simulink model "PhysicsBased_Tutorials"  (R2021a)
settings: Solver=FixedStepAuto  StartTime=0.0  StopTime=50  FixedStep=.0015  RelTol=1e-3
undefined symbols (not defined in the file): Ion, Li
libraries: PB_Library_Master x57, Lib_Solve_SSNRSolverJC_EMTAT x6, Lib_Solve_SSNRSolverJC_TMATS x1, TemperatureBlock x1
(part 1 of 2)
settings Model: Creator=nbutler2  LastModifiedBy=sfaulk
settings SolverCC: AlgebraicLoopSolver=TrustRegion
settings DebuggingCC: SFMachineParentedDataDiag=warning

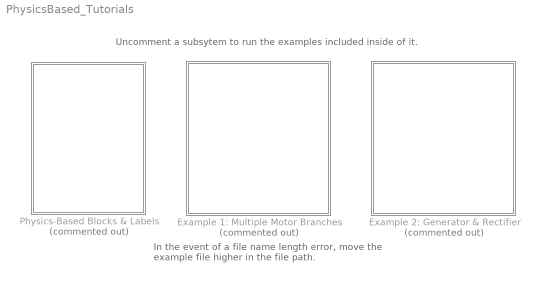
== system PhysicsBased_Tutorials ==
  note: Uncomment a subsytem to run the examples included inside of it.
  note: In the event of a file name length error, move the example file higher in the file path.
  Example 1: Multiple Motor Branches : Subsystem  Commented=on
  Example 2: Generator & Rectifier : Subsystem  Commented=on
  Physics-Based Blocks & Labels : Subsystem  Commented=on

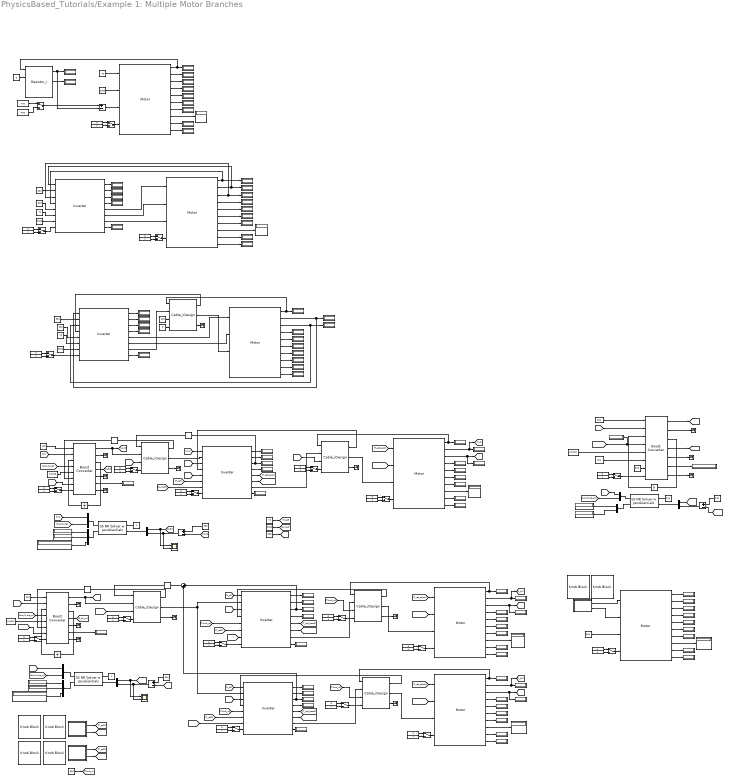
== system PhysicsBased_Tutorials/Example 1: Multiple Motor Branches ==
  note: ------------------------------------------------
      | Created by Nathan Butler
      | NASA Glenn Research Center
      | MATLAB R2020b
      | Spring 2021
      | ------------------------------------------------
  note: Current Error
  note: Solver finds solution for current input and duty cycle by driving power error (P_Err) to 0 and Vout to desired output voltage (Vdesired-Vout = 0).
  note: Model 4A: Boost Converter Example
  note: For a more detailed example, see:
      | EMTAT->Examples->Physics Based->BoostConverter_Example.m
  note: Model Inputs
  note: V_s & PF sent to inverter
  note: Some general inputs
  note: This example adds the boost converter component to the above model. A solver is used to solve for the input current and duty cycle for the boost converter. Notice that current demand is still sent backwards throughout the circuit and voltage is sent forwards.
  note: Similar to example above, but now includes cable with some small voltage loss. This example shows how the cable component can be incorporated into systems.
  note: Motor 3: Inverter-Cable-Motor Example
  note: Model 1: Current-Based Resistor-Motor Example
  note: Solves for Boost Converter input current (Iin) and duty cycle by driving P_err to zero and Vout to desired output voltage of 550V.
  note: Model includes Inverter and AC Motor. Inverter takes DC voltage input (V_batt) along with required inputs (V_s, PF, I_RMS) from motor and outputs power and current requirements (P_in_inv, I_In_inv). Mechanical properties and V_batt are passed through inverter to motor.
  note: Multi-Branch Motor Example
  note: Model 5A: Motor with Control Knobs
  note: <--- Current demanded sent backwards along top of model <---
  note: Model 4B: BoostConv-Inverter-Motor-withCables Branch
  note: Model 2: Inverter-Motor Example
  note: DC to AC
  note: DC to AC
  note: Set to desired output voltage (set point)
      | From iDesign mask window
  note: ---> Voltage sent forwards through model --->
  note: ---> Voltage sent forwards through model --->
  note: DC to AC
  note: <--- Current demanded sent backwards along top of model <---
  note: V_s & PF sent to inverter
  note: Solves for Boost Converter input current (Iin) and duty cycle by driving P_err to zero and Vout to desired output voltage of 550V.
  note: Set to desired output voltage (set point)
      | From iDesign mask window
  note: Model 5B: Multiple Motor Branch Example
  note: DC to AC
  note: DC to AC
  note: V_s & PF sent to inverter
  note: Set to:
      | (load power)/(voltage output)
      | From iDesign mask window
  note: Set to:
      | (min Vin + max Vin)/2
      | From iDesign mask window
  note: WORKS BEST WITH FIXED
      | STEP SIZE SOLVER. ENSURE
      | STEP SIZE AGREES WITH INPUT
      | TO dt ON BOOST CONVERTER
  note: Set to desired output voltage (set point)
      | From iDesign mask window
  note: Voltage Error
  note: Power Error
  note: Voltage Error
  note: Power Error
  note: Current Error
  note: Voltage Error
  note: Power Error
  note: Current Error
  note: Voltage Error
  note: Power Error
  note: Current Error
  note: Voltage Error
  note: Power Error
  note: Current Error
  note: Fault Toggle:
      | 0 is unfaulted
      | 1 is fault
  note: Fault Toggle:
      | 0 is unfaulted
      | 1 is fault
  note: Fault Toggle:
      | 0 is unfaulted
      | 1 is fault
  note: Fault Toggle:
      | 0 is unfaulted
      | 1 is fault
  note: Fault Toggle:
      | 0 is unfaulted
      | 1 is fault
  note: Fault Toggle:
      | 0 is unfaulted
      | 1 is fault
  note: Fault Toggle:
      | 0 is unfaulted
      | 1 is fault
  note: Fault Toggle:
      | 0 is unfaulted
      | 1 is fault
  note: Fault Toggle:
      | 0 is unfaulted
      | 1 is fault
  Add1 : Sum  Inputs=+-
  Add2 : Sum  Inputs=+-
  Add3 : Sum  Inputs=+-
  Boost Converter : PB_Library_Master/Boost Converter  Pdis_M=1  C_M=1.65e-07  L_M=1.7399e-05  Ron_M=0.0012  RC_M=0.037475  RL_M=0.0057739  QgTotal_M=8.6e-07  Vdiode_M=1.4  TRise_M=2.2e-08  TFall_M=8e-09  Fsw_M=250000  Vgate_M=3.5  n_MOSFET=2  MassEst_M=82.533  TempIn=Celsius  vOut=550  pow=22000  minV=110  maxV=130  rippleMode=Use defaults (5% of voltage output and 10% of inductor current)  vRip=.05  iRip=.1  freqMode=Use default frequency (250 kHz)  freq=250e3
  Boost Converter1 : PB_Library_Master/Boost Converter  Pdis_M=1  C_M=1.65e-07  L_M=1.7804e-05  Ron_M=0.0012  RC_M=0.037475  RL_M=0.0057739  QgTotal_M=8.6e-07  Vdiode_M=1.4  TRise_M=2.2e-08  TFall_M=8e-09  Fsw_M=250000  Vgate_M=3.5  n_MOSFET=2  MassEst_M=82.533  TempIn=Celsius  vOut=600  pow=22000  minV=110  maxV=130  rippleMode=Use defaults (5% of voltage output and 10% of inductor current)  vRip=.05  iRip=.1  freqMode=Use default frequency (250 kHz)  freq=250e3
  Boost Converter2 : PB_Library_Master/Boost Converter  Pdis_M=1  C_M=1.65e-07  L_M=0.00011412  Ron_M=0.0092  RC_M=0.037475  RL_M=0.03635  QgTotal_M=7.4e-08  Vdiode_M=1.4  TRise_M=7e-09  TFall_M=1e-08  Fsw_M=250000  Vgate_M=3.5  n_MOSFET=1  MassEst_M=37.515  TempIn=Celsius  vOut=540  pow=10000  minV=240  maxV=260  rippleMode=Use defaults (5% of voltage output and 10% of inductor current)  vRip=.05  iRip=.1  freqMode=Use default frequency (250 kHz)  freq=250e3
  Bus Selector1 : BusSelector  OutputSignals=Converged,JacFailed,J
  Bus Selector2 : BusSelector  OutputSignals=Converged,JacFailed,J
  Bus Selector3 : BusSelector  OutputSignals=Converged,JacFailed
  Cable_iDesign{,1..5} (6 alike) : PB_Library_Master/Cable_iDesign  rad_c_M=0.94407  t_i_M=1.0013  Mass_M=159.0996  R_init=0.006  alpha=0.00393  V_in=120  V_drop=.3  I_out=40  Len=100  FS=1.5  Mat_c=Copper  UResis=0  UDens_C=0  UAlpha=0  Mat_i=PVC  UDens_I=0  UEpsilon=0
  Constant{,5,9,14,25,42} (6 alike) : Constant  Value=528
  Constant{1,7,20,26} (4 alike) : Constant  Value=70
  Constant10 : Constant  Value=true
  Constant11 : Constant  Value=250  VectorParams1D=off  SampleTime=-1
  Constant12 : Constant  Value=120
  Constant{13,15,17,19,27,29,31,33,35,37,41,45,47,50,52,54,57,60,62,65,67} (21 alike) : Constant
  Constant16 : Constant  Value=0.0015  VectorParams1D=off
  Constant18 : Constant  Value=600
  Constant{2,8,21,39} (4 alike) : Constant  Value=3000
  Constant22 : Constant  Value=150
  Constant23 : Constant  Value=0.0015  VectorParams1D=off
  Constant{4,24,38,46} (4 alike) : Constant  Value=550
  Constant{6,28,30,32,34,36,43,48..49,51,53,55..56,58..59,61,63..64,66,68} (20 alike) : Constant  Value=0
  Constant3 : Constant  Value=5
  Constant40 : Constant  Value=120
  Constant44 : Constant  Value=0.0015  VectorParams1D=off
  Current_Final : Display
  Current_Final1 : Display
  Demux : Demux  Outputs=2
  Demux1 : Demux  Outputs=2
  Demux2 : Demux  Outputs=2
  Desired Vout : Constant  Value=540
  Display{,1..19,22..43,53..60,63..82,85..110,113..117,128..133} (107 alike) : Display
  Integrator1 : Integrator
  Integrator2 : Integrator
  Integrator3 : Integrator  InitialCondition=[0;0]
  Inverter{,1..4} (5 alike) : PB_Library_Master/Inverter  T_M=[25 175]  u_D_M=[1.16666666666667 0.999999999999998]  u_ce0_M=[0.971428571428571 0.848275862068965]  R_c_M=[0.0285714285714286 0.0551724137931034]  R_D_M=[0.0238095238095238 0.0294117647058824]  E0_M=[6.00000000000002e-05 6.00000000000002e-05]  E1_M=[5.6e-05 5.6e-05]  f_sw_M=20000  L_s_M=0.1  P_max_I=22000  V_phase_I=600  f_sw_I=0  L_s_I=0.1
  Knob : KnobBlock  ScaleMax=80
  Knob1 : KnobBlock  ScaleMax=3000
  Knob2 : KnobBlock  ScaleMax=80
  Knob3 : KnobBlock  ScaleMax=3000
  Knob4 : KnobBlock  ScaleMax=80
  Knob5 : KnobBlock  ScaleMax=3000
  Manual Switch{,1..19} (20 alike) : ManualSwitch
  Memory{1..4} (4 alike) : Memory
  Motor{,1..6} (7 alike) : PB_Library_Master/Motor  pp=2.5  flux_m=0.46219  R_s=0.032  L_s=0.00115  P_Fe_Nom=904.3614  S_nom=3000  T_nom=70  P_out_max=22000  I_max=36.5  P_in_max=30000  T_max=80  MassEst_M=136.5892  Poles_i=5  R_s_i=.032  L_s_i=.00086+0.00029  S_nom_i=3000  T_nom_i=70  P_out_max_i=22000  I_max_i=36.5  P_in_max_i=30000  K_i=121  V_nom_i=368  T_max_i=80  CalculatePFe=Compute iron losses automatically  P_Fe_Nom_i=0  I_nom_i=36.5  PF_nom_i=0.99  P_Fe_Calc_Flag=1
  Motor 1 Control : Subsystem  mask{T_ref=71.10092157679236, S_mech=2953.766794958315}
      mask Display:
      | port_label('output', 1, 'T_ref');
      | port_label('output', 2, 'S_mech');
  Motor 2 Control : Subsystem  mask{T_ref=40.40733620046448, S_mech=2126.86052952404}
      mask Display:
      | port_label('output', 1, 'T_ref');
      | port_label('output', 2, 'S_mech');
  Mux : Mux  Inputs=2
  Mux1 : Mux  Inputs=2
  Mux2 : Mux  Inputs=2
  Resistor_I : PB_Library_Master/Resistor_I  TempIn=Celsius
  SS NR Solver w JacobianCalc : Lib_Solve_SSNRSolverJC_EMTAT/SS NR Solver w JacobianCalc  SJac_Per_M=.01 * [1 -1; 1 -1]  SNR_IC_M=[1;.5]  SNR_DX_M=10  SNR_Mx_M=[100000;.99999]  SNR_Mn_M=[0.00001;.0001]  SJacobianAttempts_M=200  Cond_Limits_M=0.0001
  SS NR Solver w JacobianCalc1 : Lib_Solve_SSNRSolverJC_EMTAT/SS NR Solver w JacobianCalc  SJac_Per_M=.01 * [1 -1; 1 -1]  SNR_IC_M=[1;.5]  SNR_DX_M=10  SNR_Mx_M=[100000;.99999]  SNR_Mn_M=[0.00001;.0001]  SJacobianAttempts_M=200  Cond_Limits_M=0.0001
  SS NR Solver w JacobianCalc3 : Lib_Solve_SSNRSolverJC_EMTAT/SS NR Solver w JacobianCalc  SJac_Per_M=.01 * [1 -1; 1 -1]  SNR_IC_M=[1;.5]  SNR_DX_M=10  SNR_Mx_M=[100000;.99999]  SNR_Mn_M=[0.00001;.0001]  SJacobianAttempts_M=200  Cond_Limits_M=0.0001
  Scope1 : Scope  NumInputPorts=2
  Scope2 : Scope  NumInputPorts=2
  Subsystem5 : Subsystem  mask{T_ref=78.74341928710747, S_mech=2893.268008214925}
      mask Display:
      | port_label('output', 1, 'T_ref');
      | port_label('output', 2, 'S_mech');
  Subtract : Sum  Inputs=+-
  Sum1 : Sum  Inputs=|++
  Terminator{,1..14} (15 alike) : Terminator
  V From Source : Constant  Value=700
  V From Source1 : Constant  Value=400
  wires:
  Inverter/4 -> Display37/1
  Constant25/1 -> Inverter/5
  [S_mech] -> Inverter2/7
  Subsystem5/1(Out1) -> Motor6/1
  Inverter2/3 -> Memory1/1, Display80/1  "Current demanded by inverter is input to cable"
  Cable_iDesign3/1 -> Inverter2/4  "Current demanded by cable is input to inverter"
  Constant24/1 -> Inverter/2
  Inverter/5 -> Motor1/1  "Torque passed through inverter to motor"
  Inverter/2 -> Display39/1
  Boost Converter/1 -> Cable_iDesign2/2, [Vout]  "V from Boost Converter"
  Bus Selector1/3 -> Display98/1  "<J>"
  Inverter2/4 -> Display79/1
  [S_mech_pass] -> Motor3/2
  Motor1/1 -> Inverter/4, Display77/1  "Current demanded by motor is input to previous block"
  Constant42/1 -> [TAmb]
  Constant38/1 -> Motor6/3
  [TAmb] -> Cable_iDesign3/3
  [dutyCycle] -> Boost Converter/4
  Inverter/1 -> Display40/1
  Constant20/1 -> Inverter/6
  Boost Converter/5 -> Terminator6/1
  Bus Selector1/2 -> Display97/1  "<JacFailed>"
  Memory2/1 -> Boost Converter/6  "Current demanded by cable is input into boost converter"
  Cable_iDesign2/3 -> Terminator3/1
  SS NR Solver w JacobianCalc1/1 -> Demux/1
  Inverter/8 -> Display36/1
  Motor3/2 -> [V_s], Display93/1
  Inverter/3 -> Display38/1
  Motor1/3 -> Inverter/3, Display75/1  "Power Factor of motor is input to inverter"
  [TAmb] -> Boost Converter/7
  [T_ref] -> Inverter2/6
  Inverter/6 -> Motor1/2  "Speed passed through inverter to motor"
  [P_Err] -> Scope1/1, Mux/1
  Inverter/7 -> Motor1/3  "V_batt passed through inverter to motor"
  Boost Converter/3 -> Integrator1/1
  Motor3/9 -> Display86/1
  Subsystem5/2(Out2) -> Motor6/2
  Constant40/1 -> Boost Converter/1
  Motor1/2 -> Display76/1, Inverter/1  "Stator voltage from motor (RMS) input to inverter"
  Constant44/1 -> Boost Converter/5
  Add1/1 -> Scope1/2, Mux/2
  Boost Converter/4 -> [P_Err]
  Cable_iDesign2/1 -> Memory2/1  "Memory delay on current demand"
  Motor3/5 -> Display90/1
  Motor3/7 -> Display88/1
  Motor3/1 -> Cable_iDesign3/1, Display94/1  "Current: START HERE. Current demanded by motor is input for cable"
  Inverter2/8 -> Display68/1
  Motor3/6 -> Display89/1
  Inverter2/1 -> Display82/1
  Inverter2/2 -> Display81/1
  Constant39/1 -> [S_mech]
  Inverter2/6 -> [S_mech_pass]
  Motor3/4 -> Display91/1
  Motor3/3 -> [PF_m], Display92/1
  Motor3/8 -> Display87/1
  Motor3/10 -> Display85/1
  [V_s] -> Inverter2/1
  [TAmb] -> Cable_iDesign2/3
  [TAmb] -> Inverter2/5
  Inverter2/7 -> Cable_iDesign3/2  "V from Inverter"
  [Iin] -> Boost Converter/2
  [PF_m] -> Inverter2/3
  Constant21/1 -> Inverter/7
  SS NR Solver w JacobianCalc1/2 -> Bus Selector1/1
  Inverter2/5 -> [T_ref_pass]
  Constant26/1 -> [T_ref]
  Boost Converter/2 -> Terminator5/1
  Cable_iDesign2/2 -> Inverter2/2  "V from Cable"
  Integrator1/1 -> Boost Converter/3
  Boost Converter/7 -> Terminator7/1  "PLoss"
  Boost Converter/6 -> Current_Final/1  "Iin"
  Cable_iDesign3/3 -> Terminator4/1
  Bus Selector1/1 -> Display96/1  "<Converged>"
  Mux/1 -> SS NR Solver w JacobianCalc1/2
  [Vout] -> Add1/2
  Constant45/1 -> SS NR Solver w JacobianCalc1/1
  Constant46/1 -> Add1/1
  Demux/1 -> [Iin]
  Demux/2 -> [dutyCycle]
  Cable_iDesign3/2 -> Motor3/3  "V from Cable"
  [T_ref_pass] -> Motor3/1
  Constant3/1 -> Resistor_I/2
  Resistor_I/2 -> Display13/1
  Resistor_I/1 -> Subtract/2, Display14/1  "V drop through resistor is subtracted from source voltage"
  Manual Switch/1 -> Subtract/1
  Inverter1/3 -> Display17/1
  Cable_iDesign/2 -> Motor2/3  "V from Cable"
  Inverter1/7 -> Cable_iDesign/2  "V from Inverter"
  Motor2/8 -> Display24/1
  Motor2/10 -> Display22/1
  Cable_iDesign/3 -> Terminator1/1
  Motor2/4 -> Display35/1
  Inverter1/1 -> Display19/1
  Motor2/1 -> Cable_iDesign/1, Display55/1  "Current: START HERE. Current demanded by motor is input for cable"
  Motor2/6 -> Display33/1
  Cable_iDesign/1 -> Inverter1/4  "Current demanded by cable is input to inverter"
  Motor2/5 -> Display34/1
  Motor2/9 -> Display23/1
  Inverter1/8 -> Display15/1
  Constant6/1 -> Cable_iDesign/4
  Inverter1/2 -> Display18/1
  Inverter1/4 -> Display16/1
  Motor2/3 -> Inverter1/3, Display53/1
  Motor2/7 -> Display32/1
  Constant5/1 -> Cable_iDesign/3
  Motor2/2 -> Inverter1/1, Display54/1
  Constant4/1 -> Inverter1/2
  Inverter1/6 -> Motor2/2
  Inverter1/5 -> Motor2/1
  Constant7/1 -> Inverter1/6
  Constant8/1 -> Inverter1/7
  Constant9/1 -> Inverter1/5
  Memory1/1 -> Cable_iDesign2/1  "Current demanded by cable is input into boost converter"
  Cable_iDesign4/2 -> Motor4/3  "V from Cable"
  [dutyCycle_m] -> Boost Converter1/4
  Constant14/1 -> [TAmb_m]
  [TAmb_m] -> Cable_iDesign4/3
  Inverter3/4 -> Display57/1
  [S_mech_pass1] -> Motor4/2
  Bus Selector2/3 -> Display107/1  "<J>"
  Boost Converter1/1 -> Cable_iDesign1/2, [Vout_m]  "V from Boost Converter"
  Inverter3/3 -> Display58/1, Sum1/1  "Current demanded by inverter is input to cable"
  [S_mech1] -> Inverter3/7
  Cable_iDesign1/1 -> Memory4/1  "Memory delay on current demand"
  Motor4/10 -> Display63/1
  [TAmb_m] -> Inverter3/5
  Motor4/8 -> Display65/1
  [TAmb_m] -> Boost Converter1/7
  Motor4/6 -> Display99/1
  Motor4/7 -> Display95/1
  [Iin_m] -> Boost Converter1/2
  Constant12/1 -> Boost Converter1/1
  Boost Converter1/4 -> [P_Err_m]
  Constant16/1 -> Boost Converter1/5
  Motor4/3 -> [PF_m1], Display102/1
  Bus Selector2/2 -> Display106/1  "<JacFailed>"
  Demux1/2 -> [dutyCycle_m]
  [Vout_m] -> Add2/2
  Bus Selector2/1 -> Display105/1  "<Converged>"
  Motor4/5 -> Display100/1
  Boost Converter1/2 -> Terminator9/1
  [V_s1] -> Inverter3/1
  Motor4/1 -> Cable_iDesign4/1, Display104/1  "Current: START HERE. Current demanded by motor is input for cable"
  Cable_iDesign4/3 -> Terminator8/1
  Boost Converter1/7 -> Terminator11/1  "PLoss"
  [T_ref_pass1] -> Motor4/1
  Inverter3/1 -> Display60/1
  Motor4/4 -> Display101/1
  Cable_iDesign1/3 -> Terminator2/1
  Inverter3/7 -> Cable_iDesign4/2  "V from Inverter"
  Constant17/1 -> SS NR Solver w JacobianCalc3/1
  Inverter3/8 -> Display56/1
  [P_Err_m] -> Scope2/1, Mux1/1
  Boost Converter1/5 -> Terminator10/1
  Memory4/1 -> Boost Converter1/6  "Current demanded by cable is input into boost converter"
  Motor4/9 -> Display64/1
  [PF_m1] -> Inverter3/3
  Inverter3/6 -> [S_mech_pass1]
  [T_ref1] -> Inverter3/6
  Motor4/2 -> [V_s1], Display103/1
  Inverter3/2 -> Display59/1
  Integrator2/1 -> Boost Converter1/3
  Boost Converter1/6 -> Current_Final1/1  "Iin"
  SS NR Solver w JacobianCalc3/1 -> Demux1/1
  Demux1/1 -> [Iin_m]
  Inverter3/5 -> [T_ref_pass1]
  Constant18/1 -> Add2/1
  Add2/1 -> Scope2/2, Mux1/2
  [TAmb_m] -> Cable_iDesign1/3
  Mux1/1 -> SS NR Solver w JacobianCalc3/2
  Cable_iDesign4/1 -> Inverter3/4  "Current demanded by cable is input to inverter"
  Boost Converter1/3 -> Integrator2/1
  SS NR Solver w JacobianCalc3/2 -> Bus Selector2/1
  Cable_iDesign5/2 -> Motor5/3  "V from Cable"
  [TAmb_m] -> Cable_iDesign5/3
  Cable_iDesign5/1 -> Inverter4/4  "Current demanded by cable is input to inverter"
  Inverter4/5 -> [T_ref_pass2]
  Motor5/2 -> [V_s2], Display28/1
  Inverter4/6 -> [S_mech_pass2]
  [PF_m2] -> Inverter4/3
  Motor5/9 -> Display114/1
  Inverter4/8 -> Display30/1
  [T_ref2] -> Inverter4/6
  Inverter4/7 -> Cable_iDesign5/2  "V from Inverter"
  Inverter4/1 -> Display110/1
  [T_ref_pass2] -> Motor5/1
  Motor5/4 -> Display26/1
  Cable_iDesign1/2 -> Inverter4/2, Inverter3/2  "V from Cable"
  Cable_iDesign5/3 -> Terminator12/1
  [V_s2] -> Inverter4/1
  Motor5/5 -> Display25/1
  Motor5/3 -> [PF_m2], Display27/1
  Motor5/6 -> Display117/1
  Motor5/7 -> Display116/1
  [TAmb_m] -> Inverter4/5
  Motor5/1 -> Cable_iDesign5/1, Display29/1  "Current: START HERE. Current demanded by motor is input for cable"
  Inverter4/2 -> Display109/1
  Motor5/10 -> Display113/1
  [S_mech_pass2] -> Motor5/2
  Inverter4/4 -> Display31/1
  [S_mech2] -> Inverter4/7
  Motor5/8 -> Display115/1
  Inverter4/3 -> Display108/1, Sum1/2  "Current demanded by inverter is input to cable"
  Memory3/1 -> Cable_iDesign1/1  "Current demanded by cable is input into boost converter"
  Sum1/1 -> Memory3/1
  Motor 1 Control/1(Out1) -> [T_ref1]
  Motor 1 Control/2(Out2) -> [S_mech1]
  Motor 2 Control/1(Out1) -> [T_ref2]
  Motor 2 Control/2(Out2) -> [S_mech2]
  Motor/9 -> Display10/1
  Motor/7 -> Display5/1
  Motor/3 -> Display1/1
  Motor/10 -> Display9/1
  Motor/6 -> Display6/1
  Motor/1 -> Resistor_I/1, Display3/1  "Current demanded by motor input to resistor"
  Motor/4 -> Display8/1
  Motor/2 -> Display2/1
  Motor/8 -> Display4/1
  Motor/5 -> Display7/1
  Subtract/1 -> Motor/3
  Constant2/1 -> Motor/2
  Constant1/1 -> Motor/1
  Motor6/10 -> Display73/1
  Motor6/9 -> Display74/1
  Motor6/8 -> Display67/1
  Motor6/7 -> Display69/1
  Motor6/6 -> Display70/1
  Motor6/5 -> Display71/1
  Motor6/4 -> Display72/1
  Motor6/3 -> Display11/1
  Motor6/2 -> Display12/1
  Motor6/1 -> Display66/1
  Motor1/10 -> Display132/1
  Motor1/9 -> Display133/1
  Motor1/8 -> Display78/1
  Motor1/7 -> Display128/1
  Motor1/6 -> Display129/1
  Motor1/5 -> Display130/1
  Motor1/4 -> Display131/1
  Demux2/2 -> [dutyCycle_bc]
  Demux2/1 -> [Iin_bc]
  SS NR Solver w JacobianCalc/1 -> Demux2/1
  Mux2/1 -> SS NR Solver w JacobianCalc/2
  Constant/1 -> Boost Converter2/7
  [P_Err_bc] -> Mux2/1
  Constant10/1 -> SS NR Solver w JacobianCalc/1
  Desired Vout/1 -> Add3/1
  [Vout_bc] -> Add3/2
  Bus Selector3/1 -> Display/1  "<Converged>"
  Bus Selector3/2 -> Display41/1  "<JacFailed>"
  [dutyCycle_bc] -> Display42/1, Boost Converter2/4  "d"
  Constant11/1 -> Boost Converter2/1
  [Iin_bc] -> Boost Converter2/2
  SS NR Solver w JacobianCalc/2 -> Bus Selector3/1
  Constant23/1 -> Boost Converter2/5
  Constant22/1 -> Boost Converter2/6
  Boost Converter2/1 -> [Vout_bc]  "Vout"
  Boost Converter2/3 -> Integrator3/1
  Integrator3/1 -> Boost Converter2/3
  Boost Converter2/7 -> Terminator14/1  "PLoss"
  Boost Converter2/4 -> [P_Err_bc]
  Add3/1 -> Mux2/2
  Boost Converter2/5 -> Terminator13/1
  Boost Converter2/2 -> Terminator/1
  Boost Converter2/6 -> Display43/1  "Iin"
  V From Source/1 -> Manual Switch/1
  V From Source1/1 -> Manual Switch/2
  Constant27/1 -> Manual Switch1/2
  Manual Switch1/1 -> Motor/4
  Constant28/1 -> Manual Switch1/1
  Manual Switch2/1 -> Inverter/8
  Constant30/1 -> Manual Switch2/1
  Constant29/1 -> Manual Switch2/2
  Manual Switch3/1 -> Motor1/4
  Constant32/1 -> Manual Switch3/1
  Constant31/1 -> Manual Switch3/2
  Manual Switch4/1 -> Inverter1/8
  Constant34/1 -> Manual Switch4/1
  Constant33/1 -> Manual Switch4/2
  Manual Switch5/1 -> Boost Converter/8
  Constant36/1 -> Manual Switch5/1
  Constant35/1 -> Manual Switch5/2
  Manual Switch6/1 -> Cable_iDesign2/4
  Constant43/1 -> Manual Switch6/1
  Constant37/1 -> Manual Switch6/2
  Manual Switch7/1 -> Inverter2/8
  Constant48/1 -> Manual Switch7/1
  Constant47/1 -> Manual Switch7/2
  Manual Switch8/1 -> Cable_iDesign3/4
  Constant49/1 -> Manual Switch8/1
  Constant41/1 -> Manual Switch8/2
  Manual Switch9/1 -> Motor3/4
  Constant51/1 -> Manual Switch9/1
  Constant50/1 -> Manual Switch9/2
  Manual Switch10/1 -> Boost Converter2/8
  Constant53/1 -> Manual Switch10/1
  Constant52/1 -> Manual Switch10/2
  Manual Switch11/1 -> Boost Converter1/8
  Constant55/1 -> Manual Switch11/1
  Constant54/1 -> Manual Switch11/2
  Manual Switch12/1 -> Cable_iDesign1/4
  Constant56/1 -> Manual Switch12/1
  Constant15/1 -> Manual Switch12/2
  Manual Switch13/1 -> Inverter3/8
  Constant58/1 -> Manual Switch13/1
  Constant57/1 -> Manual Switch13/2
  Manual Switch14/1 -> Cable_iDesign4/4
  Constant59/1 -> Manual Switch14/1
  Constant13/1 -> Manual Switch14/2
  Manual Switch15/1 -> Motor4/4
  Constant61/1 -> Manual Switch15/1
  Constant60/1 -> Manual Switch15/2
  Manual Switch16/1 -> Inverter4/8
  Constant63/1 -> Manual Switch16/1
  Constant62/1 -> Manual Switch16/2
  Manual Switch17/1 -> Cable_iDesign5/4
  Constant64/1 -> Manual Switch17/1
  Constant19/1 -> Manual Switch17/2
  Manual Switch18/1 -> Motor5/4
  Constant66/1 -> Manual Switch18/1
  Constant65/1 -> Manual Switch18/2
  Manual Switch19/1 -> Motor6/4
  Constant68/1 -> Manual Switch19/1
  Constant67/1 -> Manual Switch19/2

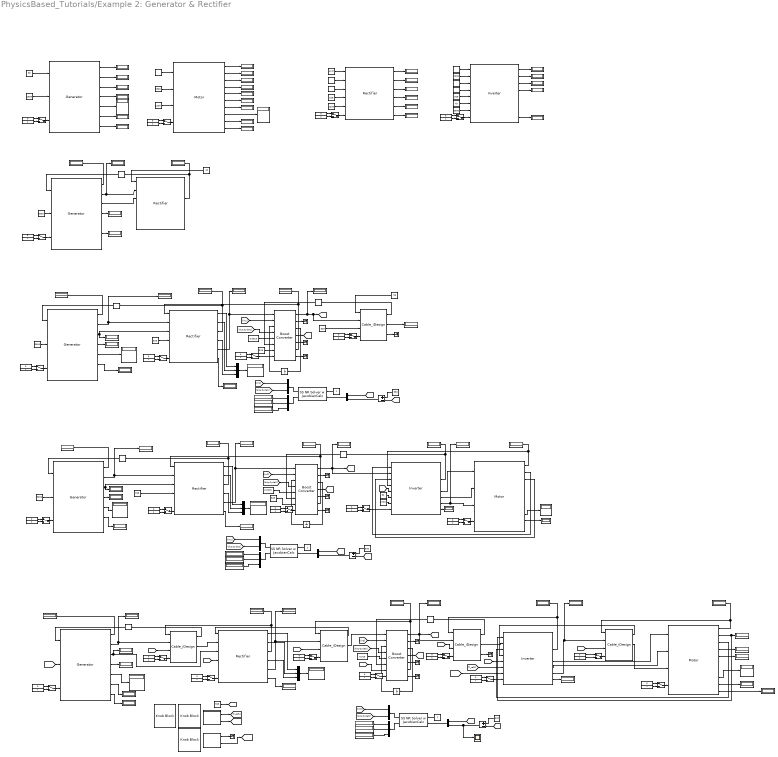
== system PhysicsBased_Tutorials/Example 2: Generator & Rectifier ==
  note: From motor
  note: These values passed to motor
  note: Model 2: Generator-Rectifier Interface
  note: Model 1B: Rectifier & Inverter Comparison
  note: Model 1A: Generator & Motor Comparison
  note: Model 3: Generator-Rectifier-BoostConverter-Cable
  note: Set to desired output voltage (set point)
      | From iDesign mask window
  note: Set to desired output voltage (set point)
      | From iDesign mask window
  note: Generator-Rectifier-BoostConverter-Inverter-Motor Full
  note: P_mechanical
  note: w_elec
  note: f_elec
  note: P_demanded
  note: Field weakening will allow generator to run past rated speed up to a point, at which the system will break.
  note: From motor
  note: From motor
  note: From generator
  note: From generator
  note: To shaft or similar block
  note: Model 4: Generator-Rectifier-BoostConverter-Inverter-Motor
  note: Set to desired output voltage (set point)
      | From iDesign mask window
  note: Model Inputs
  note: ------------------------------------------------
      | Created by Nathan Butler
      | NASA Glenn Research Center
      | MATLAB R2020b
      | Spring 2021
      | ------------------------------------------------
  note: Generator & Rectifier
  note: ---> Voltage sent forwards through model --->
  note: <--- Current demanded sent backwards along top of model <---
  note: ---> Voltage sent forwards through model --->
  note: <--- Current demanded sent backwards along top of model <---
  note: ---> Voltage sent forwards through model --->
  note: <--- Current demanded sent backwards along top of model <---
  note: Fault Toggle:
      | 0 is unfaulted
      | 1 is fault
  note: Fault Toggle:
      | 0 is unfaulted
      | 1 is fault
  note: Fault Toggle:
      | 0 is unfaulted
      | 1 is fault
  note: Fault Toggle:
      | 0 is unfaulted
      | 1 is fault
  note: Fault Toggle:
      | 0 is unfaulted
      | 1 is fault
  note: Fault Toggle:
      | 0 is unfaulted
      | 1 is fault
  note: Fault Toggle:
      | 0 is unfaulted
      | 1 is fault
  note: Fault Toggle:
      | 0 is unfaulted
      | 1 is fault
  Add1 : Sum  Inputs=+-
  Add3 : Sum  Inputs=+-
  Add6 : Sum  Inputs=+-
  Boost Converter : PB_Library_Master/Boost Converter  Pdis_M=1  C_M=1.65e-07  L_M=6.4316e-05  Ron_M=0.036  RC_M=0.037475  RL_M=0.020589  QgTotal_M=8.4e-08  Vdiode_M=1.2  TRise_M=1.72e-07  TFall_M=7.8e-08  Fsw_M=250000  Vgate_M=4  n_MOSFET=1  MassEst_M=37.515  TempIn=Celsius  vOut=550  pow=10000  minV=490  maxV=530  rippleMode=Use defaults (5% of voltage output and 10% of inductor current)  vRip=.05  iRip=.1  freqMode=Use default frequency (250 kHz)  freq=250e3
  Boost Converter3 : PB_Library_Master/Boost Converter  Pdis_M=1  C_M=1.65e-07  L_M=4.7921e-05  Ron_M=0.0092  RC_M=0.037475  RL_M=0.01523  QgTotal_M=7.4e-08  Vdiode_M=1.4  TRise_M=7e-09  TFall_M=1e-08  Fsw_M=250000  Vgate_M=3.5  n_MOSFET=1  MassEst_M=82.533  TempIn=Celsius  vOut=600  pow=22000  minV=520  maxV=550  rippleMode=Use defaults (5% of voltage output and 10% of inductor current)  vRip=.05  iRip=.1  freqMode=Use default frequency (250 kHz)  freq=250e3
  Boost Converter4 : PB_Library_Master/Boost Converter  Pdis_M=1  C_M=1.65e-07  L_M=6.4316e-05  Ron_M=0.036  RC_M=0.037475  RL_M=0.020589  QgTotal_M=8.4e-08  Vdiode_M=1.2  TRise_M=1.72e-07  TFall_M=7.8e-08  Fsw_M=250000  Vgate_M=4  n_MOSFET=1  MassEst_M=37.515  TempIn=Celsius  vOut=550  pow=10000  minV=490  maxV=530  rippleMode=Use defaults (5% of voltage output and 10% of inductor current)  vRip=.05  iRip=.1  freqMode=Use default frequency (250 kHz)  freq=250e3
  Bus Creator : BusCreator  Inputs=3
  Bus Creator1 : BusCreator  Inputs=3
  Bus Creator4 : BusCreator  Inputs=3
  Bus Selector1 : BusSelector  OutputSignals=Converged,JacFailed,J
  Bus Selector3 : BusSelector  OutputSignals=Converged,JacFailed,J
  Bus Selector6 : BusSelector  OutputSignals=Converged,JacFailed,J
  Cable_iDesign{1..3,5..6} (5 alike) : PB_Library_Master/Cable_iDesign  rad_c_M=0.94407  t_i_M=1.0013  Mass_M=159.0996  R_init=0.006  alpha=0.00393  V_in=120  V_drop=.3  I_out=40  Len=100  FS=1.5  Mat_c=Copper  UResis=0  UDens_C=0  UAlpha=0  Mat_i=PVC  UDens_I=0  UEpsilon=0
  Constant{1,4,7,15,48,67,114,120} (8 alike) : Constant  Value=528
  Constant{2,10,12,16..17,19,22,24,26..27,29,31,33..35,37,39,41,52,54,56,59,62,73,76,115} (26 alike) : Constant
  Constant{11,13,18,21,25,28,30,32,36,38,40,51,53,55,57..58,60..61,63,72,74..75,77} (23 alike) : Constant  Value=0
  Constant112 : Constant  Value=2700
  Constant113 : Constant  Value=0.0015  VectorParams1D=off
  Constant116 : Constant  Value=550
  Constant117 : Constant  Value=50
  Constant{6,69..70,119} (4 alike) : Constant  Value=3000
  Constant14 : Constant  Value=0.0015  VectorParams1D=off
  Constant20 : Constant  Value=0.015  VectorParams1D=off
  Constant23 : Constant  Value=600
  Constant3 : Constant  Value=550
  Constant42 : Constant  Value=35
  Constant43 : Constant  Value=1200
  Constant44 : Constant  Value=51.66
  Constant45 : Constant  Value=42.8
  Constant46 : Constant  Value=370.8
  Constant47 : Constant  Value=.9854
  Constant49 : Constant  Value=1200
  Constant5 : Constant  Value=36
  Constant50 : Constant  Value=370.8
  Constant64 : Constant  Value=1200
  Constant65 : Constant  Value=.9854
  Constant66 : Constant  Value=34.98
  Constant68 : Constant  Value=70
  Constant71 : Constant  Value=40
  Constant8 : Constant  Value=2500
  Constant9 : Constant  Value=2500
  Demux2 : Demux  Outputs=2
  Demux3 : Demux  Outputs=2
  Demux6 : Demux  Outputs=2
  Display{5..12,17..19,26..40,75..103,105..106,134..135,146..158} (72 alike) : Display
  Generator Control : Subsystem  mask{T_ref=71.10092157679236, S_mech=3000}
      mask Display:
      | port_label('output', 1, 'T_ref');
      | port_label('output', 2, 'S_mech');
  Generator1 : PB_Library_Master/Generator  pp=3  flux_m=0.38515  R_s=0.032  L_s=0.00115  P_Fe_Nom=904.3614  S_nom=4000  T_nom=70  P_out_max=22000  I_max=36.5  P_in_max=30000  T_max=80  MassEst_M=-1080970  Poles_i=6  R_s_i=.032  L_s_i=.00086+0.00029  S_nom_i=4000  T_nom_i=70  P_out_max_i=22000  I_max_i=36.5  P_in_max_i=30000  K_i=121  V_nom_i=368  T_max_i=80  CalculatePFe=Compute iron losses automatically  P_Fe_Nom_i=0  I_nom_i=36.5  PF_nom_i=0.99  P_Fe_Calc_Flag=1
  Generator13 : PB_Library_Master/Generator  pp=3  flux_m=0.38515  R_s=0.032  L_s=0.00115  P_Fe_Nom=904.3614  S_nom=3000  T_nom=70  P_out_max=22000  I_max=36.5  P_in_max=30000  T_max=80  MassEst_M=136.5892  Poles_i=6  R_s_i=.032  L_s_i=.00086+0.00029  S_nom_i=3000  T_nom_i=70  P_out_max_i=22000  I_max_i=36.5  P_in_max_i=30000  K_i=121  V_nom_i=368  T_max_i=80  CalculatePFe=Compute iron losses automatically  P_Fe_Nom_i=0  I_nom_i=36  PF_nom_i=0.99  P_Fe_Calc_Flag=1
  Generator2 : PB_Library_Master/Generator  pp=3  flux_m=0.38515  R_s=0.032  L_s=0.00115  P_Fe_Nom=904.3614  S_nom=4000  T_nom=70  P_out_max=22000  I_max=36.5  P_in_max=30000  T_max=80  MassEst_M=-1080970  Poles_i=6  R_s_i=.032  L_s_i=.00086+0.00029  S_nom_i=4000  T_nom_i=70  P_out_max_i=22000  I_max_i=36.5  P_in_max_i=30000  K_i=121  V_nom_i=368  T_max_i=80  CalculatePFe=Compute iron losses automatically  P_Fe_Nom_i=0  I_nom_i=36.5  PF_nom_i=0.99  P_Fe_Calc_Flag=1
  Generator3 : PB_Library_Master/Generator  pp=3  flux_m=0.38515  R_s=0.032  L_s=0.00115  P_Fe_Nom=904.3614  S_nom=3000  T_nom=70  P_out_max=22000  I_max=36.5  P_in_max=30000  T_max=80  MassEst_M=136.5892  Poles_i=6  R_s_i=.032  L_s_i=.00086+0.00029  S_nom_i=3000  T_nom_i=70  P_out_max_i=22000  I_max_i=36.5  P_in_max_i=30000  K_i=121  V_nom_i=368  T_max_i=80  CalculatePFe=Compute iron losses automatically  P_Fe_Nom_i=0  I_nom_i=36  PF_nom_i=0.99  P_Fe_Calc_Flag=1
  Generator6 : PB_Library_Master/Generator  pp=3  flux_m=0.38515  R_s=0.032  L_s=0.00115  P_Fe_Nom=904.3614  S_nom=3000  T_nom=70  P_out_max=22000  I_max=36.5  P_in_max=30000  T_max=80  MassEst_M=136.5892  Poles_i=6  R_s_i=.032  L_s_i=.00086+0.00029  S_nom_i=3000  T_nom_i=70  P_out_max_i=22000  I_max_i=36.5  P_in_max_i=30000  K_i=121  V_nom_i=368  T_max_i=80  CalculatePFe=Compute iron losses automatically  P_Fe_Nom_i=0  I_nom_i=36  PF_nom_i=0.99  P_Fe_Calc_Flag=1
  I act : Display
  Idemanded (RMS) : Display
  Idemanded (Rect) : Display
  Idemanded_BC1 : Display
  Idemanded_BC2 : Display
  Idemanded_BC5 : Display
  Idemanded_Rect : Display
  Idemanded_Rect2 : Display
  Idemanded_inv : Display
  Integrator1 : Integrator
  Integrator3 : Integrator
  Integrator6 : Integrator
  Inverter : PB_Library_Master/Inverter  T_M=[25 175]  u_D_M=[1.16666666666667 0.999999999999998]  u_ce0_M=[0.971428571428571 0.848275862068965]  R_c_M=[0.0285714285714286 0.0551724137931034]  R_D_M=[0.0238095238095238 0.0294117647058824]  E0_M=[6.00000000000002e-05 6.00000000000002e-05]  E1_M=[5.6e-05 5.6e-05]  f_sw_M=20000  L_s_M=0.1  P_max_I=22000  V_phase_I=600  f_sw_I=0  L_s_I=0.1
  Inverter1 : PB_Library_Master/Inverter  T_M=[25 175]  u_D_M=[1.16666666666667 0.999999999999998]  u_ce0_M=[0.971428571428571 0.848275862068965]  R_c_M=[0.0285714285714286 0.0551724137931034]  R_D_M=[0.0238095238095238 0.0294117647058824]  E0_M=[6.00000000000002e-05 6.00000000000002e-05]  E1_M=[5.6e-05 5.6e-05]  f_sw_M=20000  L_s_M=0.1  P_max_I=22000  V_phase_I=600  f_sw_I=0  L_s_I=0.1
  Inverter3 : PB_Library_Master/Inverter  T_M=[25 175]  u_D_M=[1.16666666666667 0.999999999999998]  u_ce0_M=[0.971428571428571 0.848275862068965]  R_c_M=[0.0285714285714286 0.0551724137931034]  R_D_M=[0.0238095238095238 0.0294117647058824]  E0_M=[6.00000000000002e-05 6.00000000000002e-05]  E1_M=[5.6e-05 5.6e-05]  f_sw_M=20000  L_s_M=0.1  P_max_I=22000  V_phase_I=600  f_sw_I=0  L_s_I=0.1
  Knob1 : KnobBlock  ScaleMax=3000
  Knob2 : KnobBlock  ScaleMax=80
  Knob3 : KnobBlock  ScaleMax=3000
  Manual Switch{1..23} (23 alike) : ManualSwitch
  Memory{1..3,5..6,12..13} (7 alike) : Memory
  Motor 1 Control : Subsystem  mask{T_ref=63.29209720829405, S_mech=2953.766794958315}
      mask Display:
      | port_label('output', 1, 'T_ref');
      | port_label('output', 2, 'S_mech');
  Motor1 : PB_Library_Master/Motor  pp=3  flux_m=0.38515  R_s=0.032  L_s=0.00115  P_Fe_Nom=904.3614  S_nom=3000  T_nom=70  P_out_max=22000  I_max=36.5  P_in_max=30000  T_max=80  MassEst_M=-1080970  Poles_i=6  R_s_i=.032  L_s_i=.00086+0.00029  S_nom_i=3000  T_nom_i=70  P_out_max_i=22000  I_max_i=36.5  P_in_max_i=30000  K_i=121  V_nom_i=368  T_max_i=80  CalculatePFe=Compute iron losses automatically  P_Fe_Nom_i=0  I_nom_i=36.5  PF_nom_i=0.99  P_Fe_Calc_Flag=1
  Motor_SI1 : PB_Library_Master/Motor  pp=3  flux_m=0.38515  R_s=0.032  L_s=0.00115  P_Fe_Nom=904.3614  S_nom=3000  T_nom=70  P_out_max=22000  I_max=36.5  P_in_max=30000  T_max=80  MassEst_M=136.5892  Poles_i=6  R_s_i=.032  L_s_i=.00086+0.00029  S_nom_i=3000  T_nom_i=70  P_out_max_i=22000  I_max_i=36.5  P_in_max_i=30000  K_i=121  V_nom_i=368  T_max_i=80  CalculatePFe=Compute iron losses automatically  P_Fe_Nom_i=0  I_nom_i=36.5  PF_nom_i=0.99  P_Fe_Calc_Flag=1
  Motor_SI4 : PB_Library_Master/Motor  pp=3  flux_m=0.38515  R_s=0.032  L_s=0.00115  P_Fe_Nom=904.3614  S_nom=3000  T_nom=70  P_out_max=22000  I_max=36.5  P_in_max=30000  T_max=80  MassEst_M=136.5892  Poles_i=6  R_s_i=.032  L_s_i=.00086+0.00029  S_nom_i=3000  T_nom_i=70  P_out_max_i=22000  I_max_i=36.5  P_in_max_i=30000  K_i=121  V_nom_i=368  T_max_i=80  CalculatePFe=Compute iron losses automatically  P_Fe_Nom_i=0  I_nom_i=36.5  PF_nom_i=0.99  P_Fe_Calc_Flag=1
  Mux2 : Mux  Inputs=2
  Mux3 : Mux  Inputs=2
  Mux6 : Mux  Inputs=2
  Rectifier{1..3,6,13} (5 alike) : PB_Library_Master/Rectifier  T_M=[25 175]  u_D_M=[1.16666666666667 0.999999999999998]  u_ce0_M=[0.971428571428571 0.848275862068965]  R_c_M=[0.0285714285714286 0.0551724137931034]  R_D_M=[0.0238095238095238 0.0294117647058824]  E0_M=[6.00000000000002e-05 6.00000000000002e-05]  E1_M=[5.6e-05 5.6e-05]  f_sw_M=20000  L_s_M=0.1  P_max_I=22000  V_phase_I=600  f_sw_I=0  L_s_I=0.1
  SS NR Solver w JacobianCalc2 : Lib_Solve_SSNRSolverJC_EMTAT/SS NR Solver w JacobianCalc  SJac_Per_M=.01 * [1 -1; 1 -1]  SNR_IC_M=[40;.5]  SNR_DX_M=5  SNR_Mx_M=[100000;.99999]  SNR_Mn_M=[0.00001;.0001]  SJacobianAttempts_M=20  Cond_Limits_M=0.0001
  SS NR Solver w JacobianCalc3 : Lib_Solve_SSNRSolverJC_EMTAT/SS NR Solver w JacobianCalc  SJac_Per_M=.01 * [1 -1; 1 -1]  SNR_IC_M=[40;.5]  SNR_DX_M=5  SNR_Mx_M=[100000;.99999]  SNR_Mn_M=[0.00001;.0001]  SJacobianAttempts_M=20  Cond_Limits_M=0.0001
  SS NR Solver w JacobianCalc6 : Lib_Solve_SSNRSolverJC_EMTAT/SS NR Solver w JacobianCalc  SJac_Per_M=.01 * [1 -1; 1 -1]  SNR_IC_M=[40;.5]  SNR_DX_M=5  SNR_Mx_M=[100000;.99999]  SNR_Mn_M=[0.00001;.0001]  SJacobianAttempts_M=20  Cond_Limits_M=0.0001
  Scope : Scope
  T_demanded : Display
  T_demanded (Gen) : Display
  T_demanded1 : Display
  T_demanded4 : Display
  Terminator{,3..6,10..13,20,25..26} (12 alike) : Terminator
  Vout (Gen) : Display
  Vout_BC1 : Display
  Vout_BC2 : Display
  Vout_BC5 : Display
  Vout_Gen (RMS) : Display
  Vout_Gen (RMS)1 : Display
  Vout_Gen (RMS)4 : Display
  Vout_Inv : Display
  Vout_Rect : Display
  Vout_Rect1 : Display
  Vout_Rect4 : Display
  wires:
  [Iin3] -> Boost Converter3/2
  Cable_iDesign3/1 -> Inverter/4
  Constant6/1 -> Generator3/2
  Motor_SI1/8 -> Display39/1
  Constant7/1 -> Boost Converter/7
  Constant3/1 -> Add3/1
  Constant5/1 -> Cable_iDesign1/1
  [TAmb] -> Inverter/5
  Motor_SI1/1 -> Display5/1, Cable_iDesign3/1
  Generator13/4 -> Display27/1
  Boost Converter3/1 -> [Vout3], Cable_iDesign2/2, Vout_BC2/1
  Inverter/8 -> Display36/1
  Generator3/4 -> Display12/1
  Constant14/1 -> Boost Converter/5
  [Iin1] -> Boost Converter/2
  Cable_iDesign2/1 -> Memory1/1
  Cable_iDesign1/2 -> Display10/1  "V from Cable"
  Boost Converter/6 -> Idemanded_BC1/1, Rectifier3/1  "Iin"
  [S_mech1] -> Inverter/7
  Rectifier13/3 -> Idemanded (RMS)/1, Cable_iDesign6/1
  Motor_SI1/3 -> Inverter/3
  Inverter/5 -> Motor_SI1/1
  Integrator1/1 -> Boost Converter3/3
  Memory2/1 -> Generator13/1
  Rectifier3/6 -> Display19/1
  Generator3/5 -> Display17/1
  Constant20/1 -> Boost Converter3/5
  Cable_iDesign6/1 -> Memory2/1
  Bus Selector3/2 -> Display8/1  "<JacFailed>"
  Boost Converter3/4 -> [P_Err3]
  [TAmb] -> Cable_iDesign2/3
  [TAmb] -> Cable_iDesign3/3
  Rectifier13/2 -> Bus Creator1/2
  Boost Converter/2 -> Terminator11/1
  Rectifier13/5 -> Cable_iDesign5/2, Vout_Rect1/1
  Boost Converter3/7 -> Terminator6/1  "PLoss"
  [TAmb] -> Cable_iDesign6/3
  Demux3/2 -> [dutyCycle3]
  [P_Err3] -> Mux3/1
  SS NR Solver w JacobianCalc3/2 -> Bus Selector1/1
  [TAmb] -> Cable_iDesign5/3
  Cable_iDesign5/2 -> Boost Converter3/1
  Cable_iDesign6/2 -> Rectifier13/2
  Generator3/6 -> Display18/1
  Generator3/3 -> Rectifier3/3, Display11/1
  Motor_SI1/9 -> Display40/1
  [T_ref1] -> Inverter/6
  Motor_SI1/4 -> Display37/1
  Cable_iDesign1/3 -> Terminator10/1
  Rectifier3/2 -> Bus Creator/2
  Inverter/7 -> Vout_Inv/1, Cable_iDesign3/2
  Cable_iDesign2/2 -> Inverter/2
  Cable_iDesign3/2 -> Motor_SI1/3
  Add1/1 -> Scope/1, Mux3/2
  Cable_iDesign2/3 -> Terminator3/1
  Generator13/6 -> Display29/1
  Rectifier13/1 -> Bus Creator1/1
  Bus Selector1/1 -> Display33/1  "<Converged>"
  SS NR Solver w JacobianCalc3/1 -> Demux3/1
  Constant23/1 -> Add1/1
  Boost Converter/4 -> [P_Err1]
  Mux3/1 -> SS NR Solver w JacobianCalc3/2
  Boost Converter3/6 -> Idemanded_BC2/1, Cable_iDesign5/1  "Iin"
  Bus Creator/1 -> Display26/1
  Constant15/1 -> Rectifier3/4
  Rectifier3/1 -> Bus Creator/1
  Rectifier3/4 -> Bus Creator/3
  Cable_iDesign1/1 -> Memory3/1
  Motor_SI1/2 -> Display35/1, Inverter/1
  Rectifier3/3 -> Idemanded_Rect/1, Memory5/1
  Demux2/1 -> [Iin1]
  Rectifier3/5 -> Vout_Rect/1, Boost Converter/1
  [P_Err1] -> Mux2/1
  Demux2/2 -> [dutyCycle1]
  Boost Converter/3 -> Integrator3/1
  Constant2/1 -> SS NR Solver w JacobianCalc2/1
  Integrator3/1 -> Boost Converter/3
  SS NR Solver w JacobianCalc2/2 -> Bus Selector3/1
  SS NR Solver w JacobianCalc2/1 -> Demux2/1
  Bus Selector3/1 -> Display7/1  "<Converged>"
  Memory3/1 -> Boost Converter/6
  Boost Converter/5 -> Terminator12/1
  Boost Converter/1 -> [Vout1], Cable_iDesign1/2, Vout_BC1/1
  Generator3/1 -> T_demanded/1
  Motor_SI1/5 -> Display38/1
  Constant4/1 -> Cable_iDesign1/3
  Add3/1 -> Mux2/2
  Demux3/1 -> [Iin3]
  [dutyCycle1] -> Boost Converter/4
  Inverter/3 -> Idemanded_inv/1, Cable_iDesign2/1
  Generator13/5 -> Display28/1
  Generator13/2 -> Cable_iDesign6/2, Vout_Gen (RMS)1/1
  [TAmb] -> Rectifier13/4
  Boost Converter3/5 -> Terminator5/1
  [Vout3] -> Add1/2
  Generator3/2 -> Rectifier3/2, Vout_Gen (RMS)/1
  Bus Creator1/1 -> Display31/1
  Constant22/1 -> SS NR Solver w JacobianCalc3/1
  Memory1/1 -> Boost Converter3/6
  Generator13/3 -> Rectifier13/3, Display9/1
  Boost Converter3/2 -> Terminator4/1
  Mux2/1 -> SS NR Solver w JacobianCalc2/2
  Cable_iDesign5/1 -> Rectifier13/1
  Generator13/1 -> T_demanded1/1
  [dutyCycle3] -> Boost Converter3/4
  Bus Selector1/3 -> Display32/1  "<J>"
  Bus Selector3/3 -> Display6/1  "<J>"
  [TAmb] -> Boost Converter3/7
  Memory5/1 -> Generator3/1
  [Vout1] -> Add3/2
  Rectifier13/4 -> Bus Creator1/3
  Bus Selector1/2 -> Display34/1  "<JacFailed>"
  Boost Converter3/3 -> Integrator1/1
  Rectifier13/6 -> Display30/1
  Boost Converter/7 -> Terminator13/1  "PLoss"
  Generator13/7 -> I act/1
  Motor_SI1/10 -> Display75/1
  Generator1/7 -> Display92/1
  Generator1/2 -> Display77/1
  Constant43/1 -> Motor1/3
  Constant42/1 -> Generator1/1
  Generator1/6 -> Display78/1
  Generator1/4 -> Display80/1
  Generator1/3 -> Display79/1
  Motor1/5 -> Display88/1
  Motor1/1 -> Display82/1  "Idemanded"
  Constant8/1 -> Generator1/2
  Constant9/1 -> Motor1/2
  Motor1/2 -> Display83/1  "V_s"
  Motor1/9 -> Display84/1
  Motor1/6 -> Display89/1
  Motor1/10 -> Display91/1  "T_EM"
  Motor1/8 -> Display87/1
  Motor1/3 -> Display85/1
  Generator1/1 -> Display76/1
  Motor1/7 -> Display90/1
  Generator1/5 -> Display81/1
  Constant44/1 -> Motor1/1  "T_ref"
  Motor1/4 -> Display86/1
  Constant49/1 -> Rectifier1/5
  Constant45/1 -> Rectifier1/1
  Rectifier1/6 -> Display98/1
  Rectifier1/3 -> Display95/1
  Rectifier1/5 -> Display97/1
  Rectifier1/2 -> Display94/1
  Constant47/1 -> Rectifier1/3
  Constant46/1 -> Rectifier1/2
  Rectifier1/4 -> Display96/1
  Constant48/1 -> Rectifier1/4
  Rectifier1/1 -> Display93/1
  Inverter1/2 -> Display100/1
  Inverter1/4 -> Display102/1
  Inverter1/3 -> Display101/1
  Constant65/1 -> Inverter1/3
  Constant50/1 -> Inverter1/1
  Inverter1/8 -> Display103/1
  Constant68/1 -> Inverter1/6
  Constant69/1 -> Inverter1/7
  Constant64/1 -> Inverter1/2
  Inverter1/1 -> Display99/1
  Constant67/1 -> Inverter1/5
  Constant66/1 -> Inverter1/4
  Generator2/1 -> T_demanded (Gen)/1
  Generator2/3 -> Rectifier2/3
  Generator2/4 -> Display105/1
  Constant70/1 -> Generator2/2
  Memory6/1 -> Generator2/1
  Generator2/2 -> Rectifier2/2, Vout (Gen)/1
  Rectifier2/3 -> Idemanded (Rect)/1, Memory6/1
  Constant71/1 -> Rectifier2/1
  Generator2/6 -> Display106/1
  Boost Converter4/7 -> Terminator26/1  "PLoss"
  [Vout2] -> Add6/2
  Memory13/1 -> Generator6/1
  Bus Selector6/3 -> Display151/1  "<J>"
  Mux6/1 -> SS NR Solver w JacobianCalc6/2
  Generator6/2 -> Vout_Gen (RMS)4/1, Rectifier6/2
  [dutyCycle2] -> Boost Converter4/4
  Add6/1 -> Mux6/2
  Generator6/1 -> T_demanded4/1
  Boost Converter4/1 -> [Vout2], Inverter3/2, Vout_BC5/1
  Boost Converter4/5 -> Terminator25/1
  Memory12/1 -> Boost Converter4/6
  Bus Selector6/1 -> Display152/1  "<Converged>"
  SS NR Solver w JacobianCalc6/1 -> Demux6/1
  SS NR Solver w JacobianCalc6/2 -> Bus Selector6/1
  Integrator6/1 -> Boost Converter4/3
  Constant115/1 -> SS NR Solver w JacobianCalc6/1
  Boost Converter4/3 -> Integrator6/1
  Demux6/2 -> [dutyCycle2]
  [P_Err2] -> Mux6/1
  Rectifier6/5 -> Vout_Rect4/1, Boost Converter4/1
  Demux6/1 -> [Iin2]
  Rectifier6/3 -> Memory13/1, Idemanded_Rect2/1
  Rectifier6/4 -> Bus Creator4/3
  Rectifier6/1 -> Bus Creator4/1
  Constant114/1 -> Rectifier6/4
  Bus Creator4/1 -> Display150/1
  Boost Converter4/4 -> [P_Err2]
  Rectifier6/2 -> Bus Creator4/2
  Generator6/3 -> Rectifier6/3, Display135/1
  Generator6/6 -> Display148/1
  Boost Converter4/2 -> Terminator20/1
  Bus Selector6/2 -> Display153/1  "<JacFailed>"
  Generator6/5 -> Display147/1
  Rectifier6/6 -> Display149/1
  Boost Converter4/6 -> Idemanded_BC5/1, Rectifier6/1  "Iin"
  [Iin2] -> Boost Converter4/2
  Constant113/1 -> Boost Converter4/5
  Generator6/4 -> Display146/1
  Constant116/1 -> Add6/1
  Constant120/1 -> Boost Converter4/7
  Constant119/1 -> Generator6/2
  Motor_SI4/9 -> Display134/1
  Inverter3/8 -> Display158/1
  Motor_SI4/8 -> Display154/1
  Constant117/1 -> Inverter3/6
  Constant112/1 -> Inverter3/7
  [Temp] -> Inverter3/5
  Inverter3/3 -> Memory12/1, Display157/1
  Inverter3/7 -> Display155/1, Motor_SI4/3
  Inverter3/6 -> Motor_SI4/2
  Inverter3/5 -> Motor_SI4/1
  Motor_SI4/1 -> Inverter3/4, Display156/1
  Motor_SI4/3 -> Inverter3/3
  Motor_SI4/2 -> Inverter3/1
  Motor 1 Control/2(Out2) -> [S_mech1]
  Motor 1 Control/1(Out1) -> [T_ref1]
  Constant1/1 -> [TAmb]
  Generator Control/1(Out1) -> Terminator/1
  Generator Control/2(Out2) -> [S_mech2]
  [S_mech2] -> Generator13/2
  Manual Switch1/1 -> Generator1/3
  Constant28/1 -> Manual Switch1/1
  Constant27/1 -> Manual Switch1/2
  Manual Switch2/1 -> Motor1/4
  Constant11/1 -> Manual Switch2/1
  Constant10/1 -> Manual Switch2/2
  Manual Switch3/1 -> Rectifier1/6
  Constant13/1 -> Manual Switch3/1
  Constant12/1 -> Manual Switch3/2
  Manual Switch4/1 -> Inverter1/8
  Constant18/1 -> Manual Switch4/1
  Constant17/1 -> Manual Switch4/2
  Manual Switch5/1 -> Generator2/3
  Constant21/1 -> Manual Switch5/1
  Constant19/1 -> Manual Switch5/2
  Manual Switch6/1 -> Generator3/3
  Constant25/1 -> Manual Switch6/1
  Constant24/1 -> Manual Switch6/2
  Manual Switch7/1 -> Rectifier3/6
  Constant30/1 -> Manual Switch7/1
  Constant26/1 -> Manual Switch7/2
  Manual Switch8/1 -> Boost Converter/8
  Constant32/1 -> Manual Switch8/1
  Constant31/1 -> Manual Switch8/2
  Manual Switch9/1 -> Cable_iDesign1/4
  Constant36/1 -> Manual Switch9/1
  Constant34/1 -> Manual Switch9/2
  Manual Switch10/1 -> Generator6/3
  Constant38/1 -> Manual Switch10/1
  Constant37/1 -> Manual Switch10/2
  Manual Switch11/1 -> Rectifier6/6
  Constant40/1 -> Manual Switch11/1
  Constant39/1 -> Manual Switch11/2
  Manual Switch12/1 -> Boost Converter4/8
  Constant51/1 -> Manual Switch12/1
  Constant41/1 -> Manual Switch12/2
  Manual Switch13/1 -> Inverter3/8
  Constant53/1 -> Manual Switch13/1
  Constant52/1 -> Manual Switch13/2
  Manual Switch14/1 -> Motor_SI4/4
  Constant55/1 -> Manual Switch14/1
  Constant54/1 -> Manual Switch14/2
  Manual Switch15/1 -> Generator13/3
  Constant57/1 -> Manual Switch15/1
  Constant56/1 -> Manual Switch15/2
  Manual Switch16/1 -> Cable_iDesign6/4
  Constant58/1 -> Manual Switch16/1
  Constant35/1 -> Manual Switch16/2
  Manual Switch17/1 -> Rectifier13/6
  Constant60/1 -> Manual Switch17/1
  Constant59/1 -> Manual Switch17/2
  Manual Switch18/1 -> Cable_iDesign5/4
  Constant61/1 -> Manual Switch18/1
  Constant33/1 -> Manual Switch18/2
  Manual Switch19/1 -> Boost Converter3/8
  Constant63/1 -> Manual Switch19/1
  Constant62/1 -> Manual Switch19/2
  Manual Switch20/1 -> Cable_iDesign2/4
  Constant72/1 -> Manual Switch20/1
  Constant16/1 -> Manual Switch20/2
  Manual Switch21/1 -> Inverter/8
  Constant74/1 -> Manual Switch21/1
  Constant73/1 -> Manual Switch21/2
  Manual Switch22/1 -> Cable_iDesign3/4
  Constant29/1 -> Manual Switch22/2
  Constant75/1 -> Manual Switch22/1
  Inverter/6 -> Motor_SI1/2
  Manual Switch23/1 -> Motor_SI1/4
  Constant76/1 -> Manual Switch23/2
  Constant77/1 -> Manual Switch23/1
